simulink model "singleBiquadTestbench"  (R2013b)
settings: Solver=ode45  StartTime=0.0  StopTime=10.0  RelTol=1e-3
undefined symbols (not defined in the file or in its folder): dfilt
libraries: dspvision x2, dsparch4 x1, dspsrcs4 x1, dspsnks4 x1
settings Model: Creator=Preben  LastModifiedBy=Preben

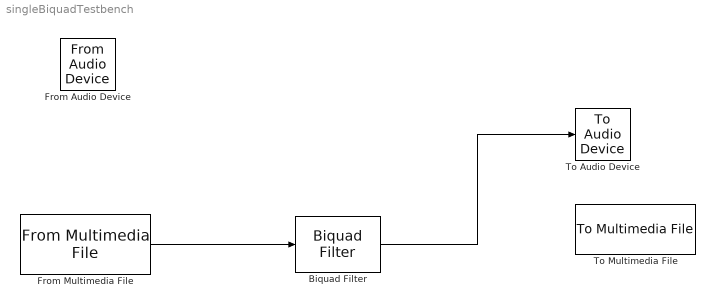
== system singleBiquadTestbench ==
  Biquad Filter : dsparch4/Biquad Filter  IIRFiltStruct=Direct form II transposed  CoeffSource=Specify via dialog  BiQuadCoeffs=[0.9069 -1.6365 0.7489 1.0000 -1.6075 0.6848]  a0Flag=Warning  IC=0  ICnum=0  ICden=0  InputProcessing=Columns as channels (frame based)  denAccumFracLength=30  denProdOutputFracLength=30  secondMemoryFracLength=15  roundingMode=Floor  overflowMode=off  ScaleValues=1  optimizeScaleValues=on  ScaleValueMode=Specify via input port (g)  scaleValueFracLength=14  FilterSource=Specify via dialog  dfiltObjectName=dfilt.df2tsos([1 0.3 0.4],[1 0.1 0.2])
  From Audio Device : dspsrcs4/From Audio Device  deviceName=ASIO Fireface USB  numChannels=1  sampleRate=44100  deviceDatatype=Determine from output data type  autoBufferSize=on  bufferSize=4096  queueDuration=1.0  frameSize=128  outputDatatype=single  defaultInputChannelMapping=off  inputChannelMapping=1:1
  From Multimedia File : dspvision/From Multimedia File  inputFilename=C:\Users\Preben\Dropbox\Matlab\Dat096\Audiofiles\07 Top Yourself_mono.wav  loop=on  numPlays=inf  outputStreams=Audio only  videoDataType=single  audioDataType=double  inheritSampleTime=on  userDefinedSampleTime=1/30  noAudioOutput=off  isIntensityVideo=off  fourcc=RGB  colorVideoFormat=Separate color signals  outputEOF=off  dataOrg=Column-major  audioFrameSize=1024  computeAudioFrameSize=off  outSamplingMode=Frame based
  To Audio Device : dspsnks4/To Audio Device  deviceName=ASIO Fireface USB  inheritSampleRate=on  sampleRate=44100  deviceDatatype=Determine from input data type  autoBufferSize=on  bufferSize=4096  queueDuration=1.0  defaultOutputChannelMapping=on  outputChannelMapping=1:18
  To Multimedia File : dspvision/To Multimedia File  outputFilename=output.wav  streamSelection=Audio only  videoCompressor=None (uncompressed)  audioCompressor=None (uncompressed)  imagePorts=Separate color signals  fileType=WAV  audioDatatype=16-bit integer  fourcc=RGB
  wires:
  From Multimedia File/1 -> Biquad Filter/1
  Biquad Filter/1 -> To Audio Device/1
